simulink model "ex_modeling_simple_system"  (R2023a)
settings: Solver=VariableStepAuto  StartTime=0.0  StopTime=10.0  RelTol=1e-3
settings Model: Creator=The MathWorks, Inc.  LastModifiedBy=grouleau
settings SolverCC: AlgebraicLoopSolver=TrustRegion
settings DataIOCC: ReturnWorkspaceOutputs=off
settings OptimizationCC: ReuseModelBlockBuffer=off
settings DebuggingCC: UnconnectedInputMsg=warning  UnconnectedOutputMsg=warning  UnconnectedLineMsg=warning  PregeneratedLibrarySubsystemCodeDiagnostic=none  ArithmeticOperatorsInVariantConditions=warning
settings ModelReferenceCC: EnableRefExpFcnMdlSchedulingChecks=on
settings SFSimCC: SimUseLocalCustomCode=off  CustomCodeUndefinedFunction=UseInterfaceOnly
settings RTWCC: RTWUseLocalCustomCode=off

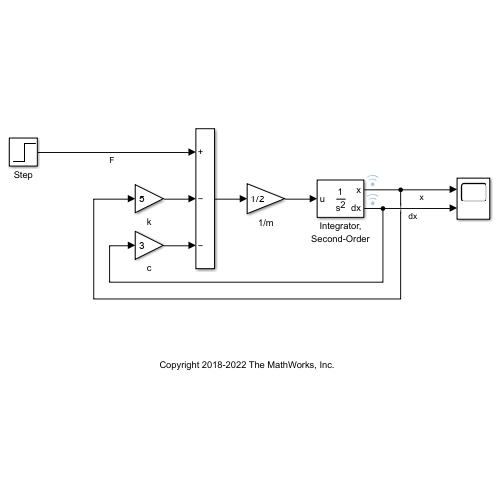
[thumbnail: Simulink's stored preview of the top-level diagram]
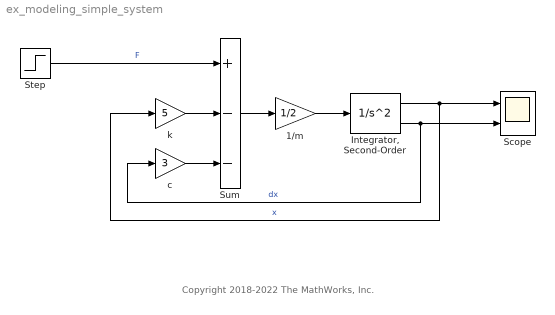
== system ex_modeling_simple_system ==
  note: Copyright 2018-2022 The MathWorks, Inc.
  1/m : Gain  Gain=1/2
  "Integrator, Second-Order" : SecondOrderIntegrator
  Scope : Scope  NumInputPorts=2
  Step : Step  SampleTime=0
  Sum : Sum  Inputs=+--
  c : Gain  Gain=3
  k : Gain  Gain=5
  wires:
  Step/1 -> Sum/1  "F"
  c/1 -> Sum/3
  k/1 -> Sum/2
  Sum/1 -> 1/m/1
  "Integrator, Second-Order"/2 -> c/1, Scope/2  "dx"
  "Integrator, Second-Order"/1 -> k/1, Scope/1  "x"
  1/m/1 -> "Integrator, Second-Order"/1
